simulink model "batteryModelSimulink"  (R2019a)
settings: Solver=VariableStepAuto  StartTime=0.0  StopTime=100  RelTol=1e-3
InitFcn:
  | load('batteryModel.mat');
  | load('soc_ocv.mat');
  | load('currentUAV.mat');
  | 
  | 
  | Q   = battery.QParam(6); % total capacity in mAh
  | n   = battery.etaParam(6); % coulombic efficiency
  | M   = battery.MParam(6); % dynamic hysteresis volts factor
  | Mo  = battery.M0Param(6); % instant hysteresis volts factor
  | Ro  = battery.R0Param(6); % internal resistance
  | R   = [battery.RCParam(6,1)]; % diffusion / warburg impedence, pairs with C
  | C   = [battery.RCParam(6,2)]; % diffusion / warburg impedence, pairs with R
  | g   = battery.GParam(6);  % gamma, tunes decay in hysteresis
  | dt  = .01; % delta t
  | 
  | if length(R) ~= length(C)
  |     error("R and C must be the same length");
  | end
  | 
  | Arc = zeros(length(R));
  | for i = 1:length(R)
  |     Arc(i,i) = exp(-dt/(R(i)*C(i)));
  | end
  | Brc = zeros(length(R), 1);
  | for i = 1:length(R)
  |     Brc(i,1) = 1 - exp(-dt/(R(i)*C(i)));
  | end
  | k = 1; % timestep
  | Io = .1; % current at time k
  | H(k) = exp(-abs((n(k)*Io(k)*g*dt)/Q));
  | 
  | 
  | Io = current(1:floor(length(current)/2.5));
  | 
  | 
  | z = 1.0; % soc
  | Ir = zeros(length(R), 1);
  | h = 0.0;
  | v = ones(length(Io));
  | 
  | 
  | soc = zeros(1, length(Io));
  | v = soc;
  | 
  | counter = 2;
  | srate = .0294
values from neighbouring files (symbols this model uses):
  battery =     [batteryModel.mat]    (also in batteryModelNew.mat)
  current = [0 0 0 0 0 0 0 0 0 0 0 0 ... (37660 elements, 1x37660)]    [current.mat]    (also in currentUAV.mat = [0 2.03088671157e-13 2.03088671157e-13 7.31118744444e-12 1.9)
  soc_ocv = [3.04 3.101 3.1589 3.2115 3.2812 3.34998 3.39958 3.46048 3.51074 3.580156 3.649925 3.7 ... (101 elements, 1x101)]    [soc_ocv_new.mat]
settings Model: Creator=tdarrah  LastModifiedBy=tdarrah

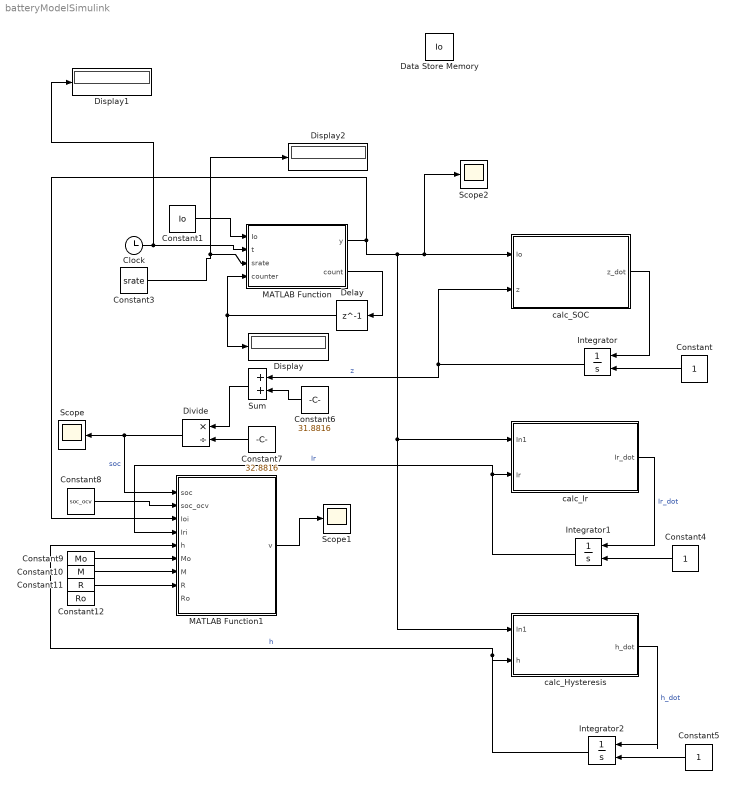
== system batteryModelSimulink ==
  Clock : Clock
  Constant : Constant
  Constant1 : Constant  Value=Io
  Constant10 : Constant  Value=M
  Constant11 : Constant  Value=R
  Constant12 : Constant  Value=Ro
  Constant3 : Constant  Value=srate
  Constant4 : Constant
  Constant5 : Constant
  Constant6 : Constant  Value=31.8816
  Constant7 : Constant  Value=32.8816
  Constant8 : Constant  Value=soc_ocv
  Constant9 : Constant  Value=Mo
  Data Store Memory : DataStoreMemory  DataStoreName=Io  ReadBeforeWriteMsg=warning  WriteAfterWriteMsg=warning  WriteAfterReadMsg=warning  ShowAdditionalParam=off
  Delay : Delay  DelayLength=1  InitialCondition=1
  Display : Display
  Display1 : Display
  Display2 : Display
  Divide : Product  Inputs=*/
  Integrator : Integrator  InitialConditionSource=external  LimitOutput=on  UpperSaturationLimit=105  LowerSaturationLimit=-5  IgnoreLimit=on
  Integrator1 : Integrator  InitialConditionSource=external  LimitOutput=on  UpperSaturationLimit=105  LowerSaturationLimit=-5  IgnoreLimit=on
  Integrator2 : Integrator  InitialConditionSource=external  LimitOutput=on  UpperSaturationLimit=105  LowerSaturationLimit=-5  IgnoreLimit=on
  MATLAB Function : MATLAB Function  TreatAsAtomicUnit=on
  MATLAB Function1 : MATLAB Function  TreatAsAtomicUnit=on
  Scope : Scope
  Scope1 : Scope
  Scope2 : Scope
  Sum : Sum
  calc_Hysteresis : Subsystem
  calc_Ir : Subsystem
  calc_SOC : Subsystem
  wires:
  MATLAB Function/1(y) -> calc_Hysteresis/1(In1), calc_Ir/1(In1), Scope2/1, calc_SOC/1(Io), MATLAB Function1/3(Ioi)
  Integrator/1 -> Sum/1, calc_SOC/2(z)  "z"
  calc_SOC/1(z_dot) -> Integrator/1
  Integrator1/1 -> calc_Ir/2(Ir), MATLAB Function1/4(Iri)  "Ir"
  calc_Ir/1(Ir_dot) -> Integrator1/1  "Ir_dot"
  calc_Hysteresis/1(h_dot) -> Integrator2/1  "h_dot"
  Constant/1 -> Integrator/2
  Clock/1 -> Display1/1, MATLAB Function/2(t)
  Constant1/1 -> MATLAB Function/1(Io)
  Delay/1 -> MATLAB Function/4(counter), Display/1
  Constant4/1 -> Integrator1/2
  Constant5/1 -> Integrator2/2
  Integrator2/1 -> MATLAB Function1/5(h), calc_Hysteresis/2(h)  "h"
  Constant6/1 -> Sum/2
  Sum/1 -> Divide/1
  Constant7/1 -> Divide/2
  Divide/1 -> MATLAB Function1/1(soc), Scope/1  "soc"
  MATLAB Function1/1(v) -> Scope1/1
  Constant8/1 -> MATLAB Function1/2(soc_ocv)
  Constant9/1 -> MATLAB Function1/6(Mo)
  Constant10/1 -> MATLAB Function1/7(M)
  Constant11/1 -> MATLAB Function1/8(R)
  Constant3/1 -> Display2/1, MATLAB Function/3(srate)
  MATLAB Function/2(count) -> Delay/1

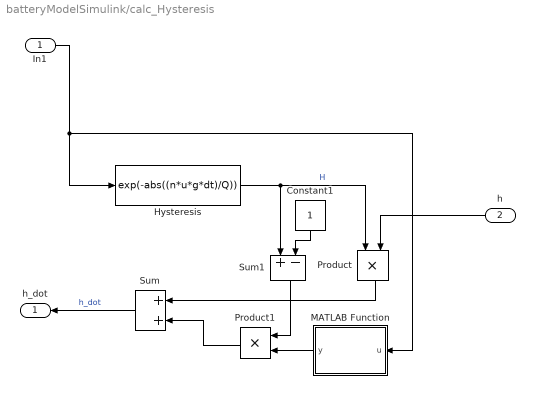
== system batteryModelSimulink/calc_Hysteresis ==
  In1 : Inport
  h : Inport  Port=2
  Constant1 : Constant
  Hysteresis : Fcn  Expr=exp(-abs((n*u*g*dt)/Q))
  MATLAB Function : MATLAB Function  TreatAsAtomicUnit=on
  Product : Product
  Product1 : Product
  Sum : Sum
  Sum1 : Sum  Inputs=+-
  h_dot : Outport
  wires:
  MATLAB Function/1(y) -> Product1/2
  h/1 -> Product/2
  In1/1 -> MATLAB Function/1(u), Hysteresis/1
  Product1/1 -> Sum/2
  Hysteresis/1 -> Sum1/1, Product/1  "H"
  Product/1 -> Sum/1
  Sum/1 -> h_dot/1  "h_dot"
  Constant1/1 -> Sum1/2
  Sum1/1 -> Product1/1

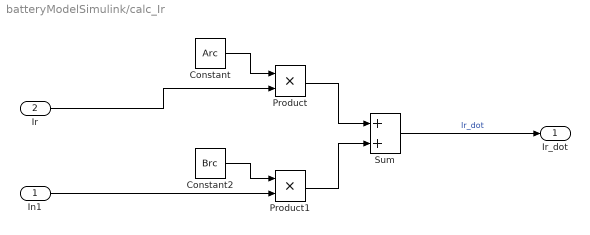
== system batteryModelSimulink/calc_Ir ==
  In1 : Inport
  Ir : Inport  Port=2
  Constant : Constant  Value=Arc
  Constant2 : Constant  Value=Brc
  Product : Product
  Product1 : Product
  Sum : Sum
  Ir_dot : Outport
  wires:
  Constant2/1 -> Product1/1
  Sum/1 -> Ir_dot/1  "Ir_dot"
  Constant/1 -> Product/1
  In1/1 -> Product1/2
  Ir/1 -> Product/2
  Product1/1 -> Sum/2
  Product/1 -> Sum/1

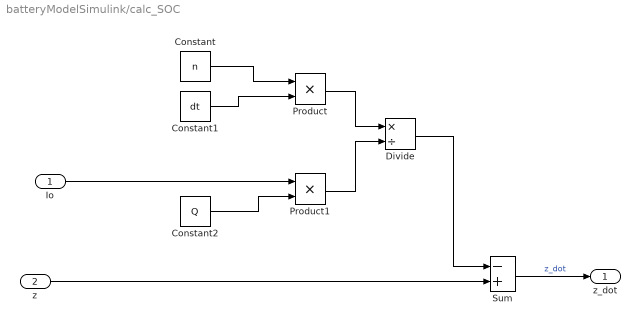
== system batteryModelSimulink/calc_SOC ==
  Io : Inport
  z : Inport  Port=2
  Constant : Constant  Value=n
  Constant1 : Constant  Value=dt
  Constant2 : Constant  Value=Q
  Divide : Product  Inputs=*/
  Product : Product
  Product1 : Product
  Sum : Sum  Inputs=-+
  z_dot : Outport
  wires:
  Divide/1 -> Sum/1
  Constant2/1 -> Product1/2
  Constant1/1 -> Product/2
  Product/1 -> Divide/1
  Constant/1 -> Product/1
  Sum/1 -> z_dot/1  "z_dot"
  Io/1 -> Product1/1
  z/1 -> Sum/2
  Product1/1 -> Divide/2

== matlab function batteryModelSimulink/MATLAB Function ==
  data: Io input; y output; t input; srate input; counter input; count output
function [y, count]= current(Io, t, srate, counter)

    if t >= counter * srate
        counter = counter + 1;
    end

    y = Io(counter);
    count = counter;

== matlab function batteryModelSimulink/calc_Hysteresis/MATLAB Function ==
  data: u input; y output
function y = sign(u)

y = sign(u(1));

== matlab function batteryModelSimulink/MATLAB Function1 ==
  data: soc input; soc_ocv input; v output; Ioi input; Iri input; h input; Mo input; M input; R input; Ro input
function v = V(soc, soc_ocv, Ioi, Iri, h, Mo, M, R, Ro)
    idx = ceil(soc*100) +1;
    v = (soc_ocv(idx) + Mo*sign(Ioi) + M*h - sum(R*Iri) - Ro*Ioi) * 3;
  %
